simulink library "MickLibBlocks"  (R2014a)
settings: Solver=ode45  StartTime=0.0  StopTime=10.0  RelTol=1e-3
values from neighbouring files (symbols this model uses):
  a = param.a    [DSC_Control_Analysis.m]    (also in DSC_Control_Analysis_Exp.m; DSC_Speed_Control_Analysis.m; EmpiricalTireCurves.m = 1.35; FFW_Fx.m = sqrt(curvature/(2*clothoidLength)))
  b = 1.15    [EmpiricalTireCurves.m]
  Cf = param.fl.C + param.fr.C    [Fyf_lookup_table.m]
  FFWax = fliplr(ax)    [FFW_Fx.m]
  m = 1724    [EmpiricalTireCurves.m]
  max_axRegen = -90*2*.91*5.5/.32/m    [FFW_Fx.m]
  maxUxRegen = max(UxRegen)    [FFW_Fx.m]
  s = 0:Step:round(sMax/Step)*Step    [FFW_Fx.m]
  Ts = 0.002    [DSC_Control_Analysis.m]    (also in DSC_Control_Analysis_Exp.m; DSC_Speed_Control_Analysis.m; EC_params_nissan.m; Ext_MPCPara.m = SSD.Ts)
  UxConstant = sqrt(mu*trackRadius*g)    [FFW_Fx.m]
undefined symbols (not defined in the file or in its folder): alphaFrontLimit, alphaRearLimit, Cr, filtera, filterb, gain_force_psi, gainFrontAlphaSlip, gainRearAlphaSlip, gainRearKappaSlip, gainRearNoneSlip, kappaFrontLimit, kappaRearLimit, lkparams, numberFIR_force, param, psi_threshold, sr, steering_limit, wc
libraries: UserBlocks x6, simulink_need_slupdate x3, MickLibBlocks x2
(part 2 of 2)

== system MickLibBlocks/ControllerP1Racing/ControllerRacingSCACS/Calculating FFW Fx/ax2volt1 ==
  ax : Inport
  Constant : Constant  Value=1.9  SampleTime=Ts
  Gear Ratio : Gain  Gain=1/5.5  SampleTime=Ts
  Sum : Sum  Inputs=|+-
  Torque2volt : Lookup  InputValues=[-90,0,210]  Table=[0,1.9,2.8]  LookUpMeth=Interpolation-Use End Values  SampleTime=Ts
  convert to force : Gain  Gain=m  SampleTime=Ts
  motor efficiency : Gain  Gain=1/.91  SampleTime=Ts
  "two motors " : Gain  Gain=1/2  SampleTime=Ts
  wheel radius : Gain  Gain=.32  SampleTime=Ts
  pedalVolt : Outport
  wires:
  ax/1 -> convert to force/1
  convert to force/1 -> wheel radius/1  "force required"
  wheel radius/1 -> Gear Ratio/1  "torque required @ wheelS"
  Gear Ratio/1 -> motor efficiency/1
  motor efficiency/1 -> "two motors "/1  "torque required  @ motorS"
  "two motors "/1 -> Torque2volt/1  "torque required  @ each motor"
  Torque2volt/1 -> Sum/1
  Sum/1 -> pedalVolt/1
  Constant/1 -> Sum/2  "remove offset as this offset will be add later in the switching logic block"

== system MickLibBlocks/ControllerP1Racing/ControllerRacingSCACS/Calculating Feedback Block/Feedback Speed ==
  GPS Vehicle State : Inport
  PostProc : Inport  Port=2
  FFWroadwheelDelta : Inport  Port=3
  SCACS : Inport  Port=4
  Bus Creator : BusCreator  Inputs=7
  Bus Selector1 : BusSelector  OutputSignals=Vx,Sideslip,Yaw Rate
  Bus Selector2 : BusSelector  OutputSignals=matchOut.deltaPsi,currentOut.currSegType
  Bus Selector3 : BusSelector  OutputSignals=Composite Steer Angle
  S-Function3 : S-Function  FunctionName=longitudinalController_psi  Parameters=psi_threshold,gain_force_psi  EnableBusSupport=off
  Weighted Moving Average : simulink_need_slupdate/Weighted Moving Average  mgainval=[ones(1,numberFIR_force)]./numberFIR_force  vinit=0.0  samptime=Ts  OutDataType=sfix(16)  OutScaling=2^-10  DoSatur=off  GainDataType=sfix( 16 )  MatRadixGroup=Best Precision: Matrix-wise  GainScaling=2^-10
  torqueFBcommand : Outport
  wires:
  Bus Selector1/1 -> Bus Creator/1  "<Vx>"
  Bus Selector1/2 -> Bus Creator/2  "<Sideslip>"
  Bus Selector1/3 -> Bus Creator/3  "<Yaw Rate>"
  FFWroadwheelDelta/1 -> Bus Creator/5
  Weighted Moving Average/1 -> torqueFBcommand/1  "torqueCommand"
  S-Function3/1 -> Weighted Moving Average/1  "torqueCommand"
  Bus Creator/1 -> S-Function3/1
  GPS Vehicle State/1 -> Bus Selector1/1
  PostProc/1 -> Bus Selector3/1
  SCACS/1 -> Bus Selector2/1
  Bus Selector2/1 -> Bus Creator/6  "<deltaPsi>"
  Bus Selector3/1 -> Bus Creator/4  "<Composite Steer Angle>"
  Bus Selector2/2 -> Bus Creator/7  "<currSegType>"

== system MickLibBlocks/ControllerP1Racing/ControllerRacingSCACS/Calculating Feedback Block/Feedback Steering Lane Keeping ==
  SCACS : Inport
  Bus Creator : BusCreator
  Bus Selector1 : BusSelector  OutputSignals=matchOut.latError,matchOut.deltaPsi
  calculate e_la : Fcn  Expr=( (a+u[3])*sin(u[2])+u[1] )*u[4]*cos(u[2])
  convert to steering at the roadwheels (rad) : Gain  Gain=-2/(param.fl.C+param.fr.C)  SaturateOnIntegerOverflow=on  OutDataTypeStr=Inherit: Same as input  ParamDataTypeStr=Inherit: Same as input
  pfk : Constant  Value=lkparams.pfk
  xla : Constant  Value=lkparams.xla
  FBroadWheelDelta : Outport
  wires:
  SCACS/1 -> Bus Selector1/1
  Bus Creator/1 -> calculate e_la/1
  pfk/1 -> Bus Creator/4
  calculate e_la/1 -> convert to steering at the roadwheels (rad)/1
  Bus Selector1/1 -> Bus Creator/1  "<latError>"
  Bus Selector1/2 -> Bus Creator/2  "<deltaPsi>"
  xla/1 -> Bus Creator/3
  convert to steering at the roadwheels (rad)/1 -> FBroadWheelDelta/1

== system MickLibBlocks/ControllerP1Racing/SwitchingLogic/Enable Logic/Delay ==
  In : Inport
  Unit Delay{,1..4} (5 alike) : UnitDelay  SampleTime=Ts
  Out : Outport
  wires:
  In/1 -> Unit Delay/1
  Unit Delay/1 -> Unit Delay1/1
  Unit Delay1/1 -> Unit Delay2/1
  Unit Delay2/1 -> Unit Delay3/1
  Unit Delay3/1 -> Unit Delay4/1
  Unit Delay4/1 -> Out/1

== system MickLibBlocks/ControllerP1Racing/SwitchingLogic/Enable Logic/Latch1 ==
  In1 : Inport
  Trigger : TriggerPort
  Out1 : Outport  InitialOutput=0
  wires:
  In1/1 -> Out1/1

== system MickLibBlocks/ControllerP1RacingError/ControllerRacingSCACS/Calculating FFW Fx/FFWstraight ==
  SCACS : Inport
  GPSvehicleState : Inport  Port=2
  Bus Selector : BusSelector  OutputSignals=Vx
  Bus Selector1 : BusSelector  OutputSignals=nextOut.nextDist,currentOut.segType
  Mux : Mux  Inputs=3
  S-Function3 : S-Function  FunctionName=FFWstraight  Parameters=max_axRegen,maxUxRegen  EnableBusSupport=off
  FFW_Fx Volt : Outport
  wires:
  Bus Selector1/2 -> Mux/3  "<segType>"
  Bus Selector1/1 -> Mux/2  "<nextDist>"
  Bus Selector/1 -> Mux/1  "<Vx>"
  Mux/1 -> S-Function3/1
  SCACS/1 -> Bus Selector1/1
  S-Function3/1 -> FFW_Fx Volt/1
  GPSvehicleState/1 -> Bus Selector/1

== system MickLibBlocks/ControllerP1RacingError/ControllerRacingSCACS/Calculating FFW Fx/ax2volt ==
  ax : Inport
  Constant : Constant  Value=1.9  SampleTime=Ts
  Gear Ratio : Gain  Gain=1/5.5  SampleTime=Ts
  Sum : Sum  Inputs=|+-
  Torque2volt : Lookup  InputValues=[-90,0,210]  Table=[0,1.9,2.8]  LookUpMeth=Interpolation-Use End Values  SampleTime=Ts
  convert to force : Gain  Gain=m  SampleTime=Ts
  motor efficiency : Gain  Gain=1/.91  SampleTime=Ts
  "two motors " : Gain  Gain=1/2  SampleTime=Ts
  wheel radius : Gain  Gain=.32  SampleTime=Ts
  pedalVolt : Outport
  wires:
  Constant/1 -> Sum/2  "remove offset as this offset will be add later in the switching logic block"
  Sum/1 -> pedalVolt/1
  Torque2volt/1 -> Sum/1
  "two motors "/1 -> Torque2volt/1  "torque required  @ each motor"
  motor efficiency/1 -> "two motors "/1  "torque required  @ motorS"
  Gear Ratio/1 -> motor efficiency/1
  wheel radius/1 -> Gear Ratio/1  "torque required @ wheelS"
  convert to force/1 -> wheel radius/1  "force required"
  ax/1 -> convert to force/1

== system MickLibBlocks/ControllerP1RacingError/ControllerRacingSCACS/Calculating FFW Fx/ax2volt1 ==
  ax : Inport
  Constant : Constant  Value=1.9  SampleTime=Ts
  Gear Ratio : Gain  Gain=1/5.5  SampleTime=Ts
  Sum : Sum  Inputs=|+-
  Torque2volt : Lookup  InputValues=[-90,0,210]  Table=[0,1.9,2.8]  LookUpMeth=Interpolation-Use End Values  SampleTime=Ts
  convert to force : Gain  Gain=m  SampleTime=Ts
  motor efficiency : Gain  Gain=1/.91  SampleTime=Ts
  "two motors " : Gain  Gain=1/2  SampleTime=Ts
  wheel radius : Gain  Gain=.32  SampleTime=Ts
  pedalVolt : Outport
  wires:
  Constant/1 -> Sum/2  "remove offset as this offset will be add later in the switching logic block"
  Sum/1 -> pedalVolt/1
  Torque2volt/1 -> Sum/1
  "two motors "/1 -> Torque2volt/1  "torque required  @ each motor"
  motor efficiency/1 -> "two motors "/1  "torque required  @ motorS"
  Gear Ratio/1 -> motor efficiency/1
  wheel radius/1 -> Gear Ratio/1  "torque required @ wheelS"
  convert to force/1 -> wheel radius/1  "force required"
  ax/1 -> convert to force/1

== system MickLibBlocks/ControllerP1RacingError/ControllerRacingSCACS/Calculating Feedback Block/Feedback Fx ==
  GPS Vehicle State : Inport
  tireSlips : Inport  Port=2
  FBroadWheelDeltaSlipLimited : Inport  Port=3
  SCACS : Inport  Port=4
  Bus Creator : BusCreator  Inputs=8
  Bus Creator1 : BusCreator
  Bus Selector1 : BusSelector  OutputSignals=Vx
  Bus Selector2 : BusSelector  OutputSignals=alphaFront,alphaRear,kappaFront,kappaRear
  Bus Selector3 : BusSelector  OutputSignals=currentOut.segType
  Constant : Constant  Value=alphaFrontLimit  SampleTime=Ts
  Constant1 : Constant  Value=alphaRearLimit  SampleTime=Ts
  Constant2 : Constant  Value=kappaFrontLimit  SampleTime=Ts
  Constant3 : Constant  Value=kappaRearLimit  SampleTime=Ts
  S-Function3 : S-Function  FunctionName=longitudinalControllerSlipCircle  Parameters=gainFrontAlphaSlip,gainRearKappaSlip,gainRearAlphaSlip,gainRearNoneSlip  EnableBusSupport=off
  Weighted Moving Average : simulink_need_slupdate/Weighted Moving Average  mgainval=[ones(1,numberFIR_force)]./numberFIR_force  vinit=0.0  samptime=Ts  OutDataType=sfix(16)  OutScaling=2^-10  DoSatur=off  GainDataType=sfix( 16 )  MatRadixGroup=Best Precision: Matrix-wise  GainScaling=2^-10
  forceFBcommand : Outport
  wires:
  GPS Vehicle State/1 -> Bus Selector1/1
  Bus Creator/1 -> S-Function3/1
  S-Function3/1 -> Weighted Moving Average/1  "forceCommand"
  Weighted Moving Average/1 -> forceFBcommand/1  "forceCommand"
  Bus Selector1/1 -> Bus Creator/1  "<Vx>"
  tireSlips/1 -> Bus Selector2/1
  Bus Selector2/1 -> Bus Creator/2  "<alphaFront>"
  Bus Selector2/2 -> Bus Creator/3  "<alphaRear>"
  Bus Selector2/3 -> Bus Creator/4  "<kappaFront>"
  Bus Selector2/4 -> Bus Creator/5  "<kappaRear>"
  FBroadWheelDeltaSlipLimited/1 -> Bus Creator/6
  SCACS/1 -> Bus Selector3/1
  Bus Selector3/1 -> Bus Creator/7  "<segType>"
  Constant/1 -> Bus Creator1/1
  Constant1/1 -> Bus Creator1/2
  Constant2/1 -> Bus Creator1/3
  Constant3/1 -> Bus Creator1/4
  Bus Creator1/1 -> Bus Creator/8

== system MickLibBlocks/ControllerP1RacingError/ControllerRacingSCACS/Calculating Feedback Block/Feedback Steering Lane Keeping ==
  SCACS : Inport
  Bus Creator : BusCreator
  Bus Selector1 : BusSelector  OutputSignals=currentOut.latError,currentOut.deltaPsi
  calculate e_la : Fcn  Expr=( (a+u[3])*sin(u[2])+u[1] )*u[4]*cos(u[2])
  convert to steering at the roadwheels (rad) : Gain  Gain=-2/(param.fl.C+param.fr.C)  SaturateOnIntegerOverflow=on  OutDataTypeStr=Inherit: Same as input  ParamDataTypeStr=Inherit: Same as input
  pfk : Constant  Value=lkparams.pfk
  xla : Constant  Value=lkparams.xla
  FBroadWheelDelta : Outport
  wires:
  convert to steering at the roadwheels (rad)/1 -> FBroadWheelDelta/1
  xla/1 -> Bus Creator/3
  Bus Selector1/2 -> Bus Creator/2  "<deltaPsi>"
  Bus Selector1/1 -> Bus Creator/1  "<latError>"
  calculate e_la/1 -> convert to steering at the roadwheels (rad)/1
  pfk/1 -> Bus Creator/4
  Bus Creator/1 -> calculate e_la/1
  SCACS/1 -> Bus Selector1/1

== system MickLibBlocks/ControllerP1RacingError/ControllerRacingSCACS/Calculating Feedback Block/calculateSlips ==
  GPS Vehicle State : Inport
  PostProc : Inport  Port=2
  Bus Creator : BusCreator  Inputs=6
  Bus Creator1 : BusCreator
  Bus Selector1 : BusSelector  OutputSignals=Sideslip,Yaw Rate,Vx
  Bus Selector2 : BusSelector  OutputSignals=Composite Steer Angle
  Bus Selector3 : BusSelector  OutputSignals=Front Wheel Speeds,Rear Wheel Speeds
  Butterworth Filter1 : DiscreteFilter  Numerator=filterb  Denominator=filtera  SampleTime=Ts
  Butterworth Filter2 : DiscreteFilter  Numerator=filterb  Denominator=filtera  SampleTime=Ts
  Demux : Demux
  S-Function3 : S-Function  FunctionName=tireSlip  Parameters=a,b  EnableBusSupport=off
  average together1 : Gain  Gain=[0.5 0.5]  Multiplication=Matrix(K*u)
  average together2 : Gain  Gain=[0.5 0.5]  Multiplication=Matrix(K*u)
  rev/s to m/s1 : Gain  Gain=[param.fl.r ; param.fr.r]*2*pi
  rev/s to m/s2 : Gain  Gain=[param.fl.r ; param.fr.r]*2*pi
  ticks/sample to rev/s1 : Gain  Gain="1/(48*2)  *  1/Ts"
  ticks/sample to rev/s2 : Gain  Gain="1/(48*2)  *  1/Ts"
  tireSlips : Outport
  wires:
  GPS Vehicle State/1 -> Bus Selector1/1
  PostProc/1 -> Bus Selector2/1
  Bus Creator/1 -> S-Function3/1
  Bus Selector1/1 -> Bus Creator/1  "<Sideslip>"
  Bus Selector1/2 -> Bus Creator/2  "<Yaw Rate>"
  Bus Selector1/3 -> Bus Creator/3  "<Vx>"
  Bus Selector2/1 -> Bus Creator/4  "<Composite Steer Angle>"
  S-Function3/1 -> Demux/1
  Demux/1 -> Bus Creator1/1  "alphaFront"
  Demux/2 -> Bus Creator1/2  "alphaRear"
  Demux/3 -> Bus Creator1/3  "kappaFront"
  Demux/4 -> Bus Creator1/4  "kappaRear"
  Bus Creator1/1 -> tireSlips/1
  ticks/sample to rev/s1/1 -> rev/s to m/s1/1
  rev/s to m/s1/1 -> average together1/1
  average together1/1 -> Butterworth Filter1/1
  Butterworth Filter1/1 -> Bus Creator/5  "front wheel speed"
  ticks/sample to rev/s2/1 -> rev/s to m/s2/1
  rev/s to m/s2/1 -> average together2/1
  average together2/1 -> Butterworth Filter2/1
  Butterworth Filter2/1 -> Bus Creator/6  "rear wheel speed"
  [global_Wheelspeeds] -> Bus Selector3/1
  Bus Selector3/1 -> ticks/sample to rev/s1/1  "<Front Wheel Speeds>"
  Bus Selector3/2 -> ticks/sample to rev/s2/1  "<Rear Wheel Speeds>"

== system MickLibBlocks/ControllerP1RacingError/SwitchingLogic/Enable Logic/Delay ==
  In : Inport
  Unit Delay{,1..4} (5 alike) : UnitDelay  SampleTime=Ts
  Out : Outport
  wires:
  Unit Delay4/1 -> Out/1
  Unit Delay3/1 -> Unit Delay4/1
  Unit Delay2/1 -> Unit Delay3/1
  Unit Delay1/1 -> Unit Delay2/1
  Unit Delay/1 -> Unit Delay1/1
  In/1 -> Unit Delay/1

== system MickLibBlocks/ControllerP1RacingError/SwitchingLogic/Enable Logic/Latch1 ==
  In1 : Inport
  Trigger : TriggerPort
  Out1 : Outport  InitialOutput=0
  wires:
  In1/1 -> Out1/1

== system MickLibBlocks/ControllerP1RacingSlipCircle/ControllerRacingSlipCircle/Calculating FFW Fx/FFWstraight ==
  SCACS : Inport
  GPSvehicleState : Inport  Port=2
  Bus Selector : BusSelector  OutputSignals=Vx
  Bus Selector1 : BusSelector  OutputSignals=nextOut.nextDist,currentOut.segType
  Mux : Mux  Inputs=3
  S-Function3 : S-Function  FunctionName=FFWstraight  Parameters=max_axRegen,maxUxRegen  EnableBusSupport=off
  FFW_Fx Volt : Outport
  wires:
  GPSvehicleState/1 -> Bus Selector/1
  S-Function3/1 -> FFW_Fx Volt/1
  SCACS/1 -> Bus Selector1/1
  Mux/1 -> S-Function3/1
  Bus Selector/1 -> Mux/1  "<Vx>"
  Bus Selector1/1 -> Mux/2  "<nextDist>"
  Bus Selector1/2 -> Mux/3  "<segType>"

== system MickLibBlocks/ControllerP1RacingSlipCircle/ControllerRacingSlipCircle/Calculating FFW Fx/ax2volt ==
  ax : Inport
  Constant : Constant  Value=1.9  SampleTime=Ts
  Gear Ratio : Gain  Gain=1/5.5  SampleTime=Ts
  Sum : Sum  Inputs=|+-
  Torque2volt : Lookup  InputValues=[-90,0,210]  Table=[0,1.9,2.8]  LookUpMeth=Interpolation-Use End Values  SampleTime=Ts
  convert to force : Gain  Gain=m  SampleTime=Ts
  motor efficiency : Gain  Gain=1/.91  SampleTime=Ts
  "two motors " : Gain  Gain=1/2  SampleTime=Ts
  wheel radius : Gain  Gain=.32  SampleTime=Ts
  pedalVolt : Outport
  wires:
  ax/1 -> convert to force/1
  convert to force/1 -> wheel radius/1  "force required"
  wheel radius/1 -> Gear Ratio/1  "torque required @ wheelS"
  Gear Ratio/1 -> motor efficiency/1
  motor efficiency/1 -> "two motors "/1  "torque required  @ motorS"
  "two motors "/1 -> Torque2volt/1  "torque required  @ each motor"
  Torque2volt/1 -> Sum/1
  Sum/1 -> pedalVolt/1
  Constant/1 -> Sum/2  "remove offset as this offset will be add later in the switching logic block"

== system MickLibBlocks/ControllerP1RacingSlipCircle/ControllerRacingSlipCircle/Calculating FFW Fx/ax2volt1 ==
  ax : Inport
  Constant : Constant  Value=1.9  SampleTime=Ts
  Gear Ratio : Gain  Gain=1/5.5  SampleTime=Ts
  Sum : Sum  Inputs=|+-
  Torque2volt : Lookup  InputValues=[-90,0,210]  Table=[0,1.9,2.8]  LookUpMeth=Interpolation-Use End Values  SampleTime=Ts
  convert to force : Gain  Gain=m  SampleTime=Ts
  motor efficiency : Gain  Gain=1/.91  SampleTime=Ts
  "two motors " : Gain  Gain=1/2  SampleTime=Ts
  wheel radius : Gain  Gain=.32  SampleTime=Ts
  pedalVolt : Outport
  wires:
  ax/1 -> convert to force/1
  convert to force/1 -> wheel radius/1  "force required"
  wheel radius/1 -> Gear Ratio/1  "torque required @ wheelS"
  Gear Ratio/1 -> motor efficiency/1
  motor efficiency/1 -> "two motors "/1  "torque required  @ motorS"
  "two motors "/1 -> Torque2volt/1  "torque required  @ each motor"
  Torque2volt/1 -> Sum/1
  Sum/1 -> pedalVolt/1
  Constant/1 -> Sum/2  "remove offset as this offset will be add later in the switching logic block"

== system MickLibBlocks/ControllerP1RacingSlipCircle/ControllerRacingSlipCircle/Calculating Feedback Block/Feedback Fx ==
  GPS Vehicle State : Inport
  tireSlips : Inport  Port=2
  FBroadWheelDeltaSlipLimited : Inport  Port=3
  SCACS : Inport  Port=4
  Bus Creator : BusCreator  Inputs=8
  Bus Creator1 : BusCreator
  Bus Selector1 : BusSelector  OutputSignals=Vx
  Bus Selector2 : BusSelector  OutputSignals=alphaFront,alphaRear,kappaFront,kappaRear
  Bus Selector3 : BusSelector  OutputSignals=currentOut.segType
  Constant : Constant  Value=alphaFrontLimit  SampleTime=Ts
  Constant1 : Constant  Value=alphaRearLimit  SampleTime=Ts
  Constant2 : Constant  Value=kappaFrontLimit  SampleTime=Ts
  Constant3 : Constant  Value=kappaRearLimit  SampleTime=Ts
  S-Function3 : S-Function  FunctionName=longitudinalControllerSlipCircleAlphaOnly  Parameters=gainFrontAlphaSlip,gainRearKappaSlip,gainRearAlphaSlip,gainRearNoneSlip  EnableBusSupport=off
  Weighted Moving Average : simulink_need_slupdate/Weighted Moving Average  mgainval=[ones(1,numberFIR_force)]./numberFIR_force  vinit=0.0  samptime=Ts  OutDataType=sfix(16)  OutScaling=2^-10  DoSatur=off  GainDataType=sfix( 16 )  MatRadixGroup=Best Precision: Matrix-wise  GainScaling=2^-10
  forceFBcommand : Outport
  wires:
  Bus Creator1/1 -> Bus Creator/8
  Constant3/1 -> Bus Creator1/4
  Constant2/1 -> Bus Creator1/3
  Constant1/1 -> Bus Creator1/2
  Constant/1 -> Bus Creator1/1
  Bus Selector3/1 -> Bus Creator/7  "<segType>"
  SCACS/1 -> Bus Selector3/1
  FBroadWheelDeltaSlipLimited/1 -> Bus Creator/6
  Bus Selector2/4 -> Bus Creator/5  "<kappaRear>"
  Bus Selector2/3 -> Bus Creator/4  "<kappaFront>"
  Bus Selector2/2 -> Bus Creator/3  "<alphaRear>"
  Bus Selector2/1 -> Bus Creator/2  "<alphaFront>"
  tireSlips/1 -> Bus Selector2/1
  Bus Selector1/1 -> Bus Creator/1  "<Vx>"
  Weighted Moving Average/1 -> forceFBcommand/1  "forceCommand"
  S-Function3/1 -> Weighted Moving Average/1  "forceCommand"
  Bus Creator/1 -> S-Function3/1
  GPS Vehicle State/1 -> Bus Selector1/1

== system MickLibBlocks/ControllerP1RacingSlipCircle/ControllerRacingSlipCircle/Calculating Feedback Block/Feedback Steering Lane Keeping ==
  SCACS : Inport
  Bus Creator : BusCreator
  Bus Selector1 : BusSelector  OutputSignals=currentOut.latError,currentOut.deltaPsi
  calculate e_la : Fcn  Expr=( (a+u[3])*sin(u[2])+u[1] )*u[4]*cos(u[2])
  convert to steering at the roadwheels (rad) : Gain  Gain=-2/(param.fl.C+param.fr.C)  SaturateOnIntegerOverflow=on  OutDataTypeStr=Inherit: Same as input  ParamDataTypeStr=Inherit: Same as input
  pfk : Constant  Value=lkparams.pfk
  xla : Constant  Value=lkparams.xla
  FBroadWheelDelta : Outport
  wires:
  SCACS/1 -> Bus Selector1/1
  Bus Creator/1 -> calculate e_la/1
  pfk/1 -> Bus Creator/4
  calculate e_la/1 -> convert to steering at the roadwheels (rad)/1
  Bus Selector1/1 -> Bus Creator/1  "<latError>"
  Bus Selector1/2 -> Bus Creator/2  "<deltaPsi>"
  xla/1 -> Bus Creator/3
  convert to steering at the roadwheels (rad)/1 -> FBroadWheelDelta/1

== system MickLibBlocks/ControllerP1RacingSlipCircle/ControllerRacingSlipCircle/Calculating Feedback Block/Feedback Steering Limit Slip ==
  tireSlips : Inport
  Bus Creator : BusCreator  Inputs=2
  Bus Selector1 : BusSelector  OutputSignals=alphaFront
  Constant : Constant  Value=alphaFrontLimit  SampleTime=Ts
  S-Function3 : S-Function  FunctionName=FBsteeringLimitAlpha  EnableBusSupport=off
  FBroadWheelDeltaSlipLimited : Outport
  wires:
  Bus Creator/1 -> S-Function3/1
  Constant/1 -> Bus Creator/2
  Bus Selector1/1 -> Bus Creator/1  "<alphaFront>"
  tireSlips/1 -> Bus Selector1/1
  S-Function3/1 -> FBroadWheelDeltaSlipLimited/1

== system MickLibBlocks/ControllerP1RacingSlipCircle/ControllerRacingSlipCircle/Calculating Feedback Block/calculateSlips ==
  GPS Vehicle State : Inport
  PostProc : Inport  Port=2
  Bus Creator : BusCreator  Inputs=6
  Bus Creator1 : BusCreator
  Bus Selector1 : BusSelector  OutputSignals=Sideslip,Yaw Rate,Vx
  Bus Selector2 : BusSelector  OutputSignals=Composite Steer Angle
  Bus Selector3 : BusSelector  OutputSignals=Front Wheel Speeds,Rear Wheel Speeds
  Butterworth Filter1 : DiscreteFilter  Numerator=filterb  Denominator=filtera  SampleTime=Ts
  Butterworth Filter2 : DiscreteFilter  Numerator=filterb  Denominator=filtera  SampleTime=Ts
  Demux : Demux
  S-Function3 : S-Function  FunctionName=tireSlip  Parameters=a,b  EnableBusSupport=off
  average together1 : Gain  Gain=[0.5 0.5]  Multiplication=Matrix(K*u)
  average together2 : Gain  Gain=[0.5 0.5]  Multiplication=Matrix(K*u)
  rev/s to m/s1 : Gain  Gain=[param.fl.r ; param.fr.r]*2*pi
  rev/s to m/s2 : Gain  Gain=[param.fl.r ; param.fr.r]*2*pi
  ticks/sample to rev/s1 : Gain  Gain="1/(48*2)  *  1/Ts"
  ticks/sample to rev/s2 : Gain  Gain="1/(48*2)  *  1/Ts"
  tireSlips : Outport
  wires:
  Bus Selector3/2 -> ticks/sample to rev/s2/1  "<Rear Wheel Speeds>"
  Bus Selector3/1 -> ticks/sample to rev/s1/1  "<Front Wheel Speeds>"
  [global_Wheelspeeds] -> Bus Selector3/1
  Butterworth Filter2/1 -> Bus Creator/6  "rear wheel speed"
  average together2/1 -> Butterworth Filter2/1
  rev/s to m/s2/1 -> average together2/1
  ticks/sample to rev/s2/1 -> rev/s to m/s2/1
  Butterworth Filter1/1 -> Bus Creator/5  "front wheel speed"
  average together1/1 -> Butterworth Filter1/1
  rev/s to m/s1/1 -> average together1/1
  ticks/sample to rev/s1/1 -> rev/s to m/s1/1
  Bus Creator1/1 -> tireSlips/1
  Demux/4 -> Bus Creator1/4  "kappaRear"
  Demux/3 -> Bus Creator1/3  "kappaFront"
  Demux/2 -> Bus Creator1/2  "alphaRear"
  Demux/1 -> Bus Creator1/1  "alphaFront"
  S-Function3/1 -> Demux/1
  Bus Selector2/1 -> Bus Creator/4  "<Composite Steer Angle>"
  Bus Selector1/3 -> Bus Creator/3  "<Vx>"
  Bus Selector1/2 -> Bus Creator/2  "<Yaw Rate>"
  Bus Selector1/1 -> Bus Creator/1  "<Sideslip>"
  Bus Creator/1 -> S-Function3/1
  PostProc/1 -> Bus Selector2/1
  GPS Vehicle State/1 -> Bus Selector1/1

== system MickLibBlocks/ControllerP1RacingSlipCircle/SwitchingLogic/Enable Logic/Delay ==
  In : Inport
  Unit Delay{,1..4} (5 alike) : UnitDelay  SampleTime=Ts
  Out : Outport
  wires:
  In/1 -> Unit Delay/1
  Unit Delay/1 -> Unit Delay1/1
  Unit Delay1/1 -> Unit Delay2/1
  Unit Delay2/1 -> Unit Delay3/1
  Unit Delay3/1 -> Unit Delay4/1
  Unit Delay4/1 -> Out/1

== system MickLibBlocks/ControllerP1RacingSlipCircle/SwitchingLogic/Enable Logic/Latch1 ==
  In1 : Inport
  Trigger : TriggerPort
  Out1 : Outport  InitialOutput=0
  wires:
  In1/1 -> Out1/1
